simulink model "ysw11_17"  (R2014a)
settings: Solver=ode45  StartTime=0.0  StopTime=10.0  RelTol=1e-3
libraries: commdigbbndfm2 x1
settings Model: Creator=ii  LastModifiedBy=ii
settings SolverCC: ZeroCrossAlgorithm=Adaptive
settings DebuggingCC: UnderspecifiedInitializationDetection=Classic

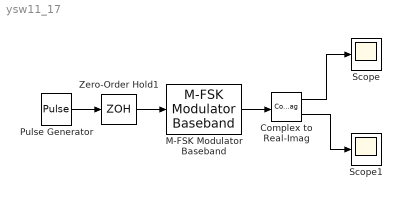
== system ysw11_17 ==
  Complex to Real-Imag : ComplexToRealImag
  M-FSK Modulator Baseband : commdigbbndfm2/M-FSK Modulator Baseband  M=8  InType=Integer  Enc=Gray  freqSep=6  phaseType=Continuous  numSamp=17  RateOptions=Enforce single-rate processing  outDataType=double
  Pulse Generator : DiscretePulseGenerator  PulseType=Time based  Amplitude=3  Period=10  PulseWidth=5
  Scope : Scope
  Scope1 : Scope
  Zero-Order Hold1 : ZeroOrderHold
  wires:
  Pulse Generator/1 -> Zero-Order Hold1/1
  Zero-Order Hold1/1 -> M-FSK Modulator Baseband/1
  M-FSK Modulator Baseband/1 -> Complex to Real-Imag/1
  Complex to Real-Imag/1 -> Scope/1
  Complex to Real-Imag/2 -> Scope1/1
